simulink model "simulink_caso3_digital"  (R2023a)
settings: Solver=VariableStepAuto  StartTime=0.0  StopTime=10.0  RelTol=1e-3
undefined symbols (not defined in the file): Ad, Aestd, Bd, Bestd, Cd, Cestd, Dd, Destd, K00d, Ts
settings Model: Creator=Agustin  LastModifiedBy=Agustin

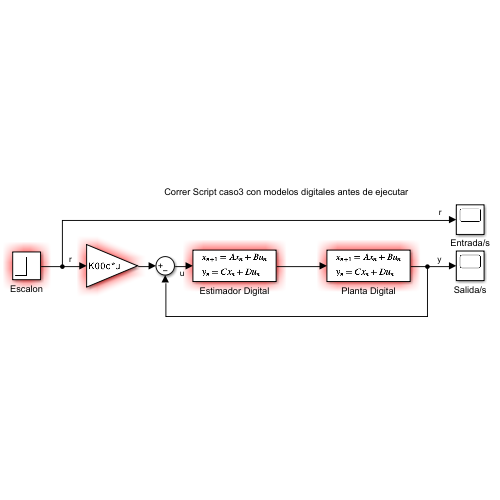
[thumbnail: Simulink's stored preview of the top-level diagram]
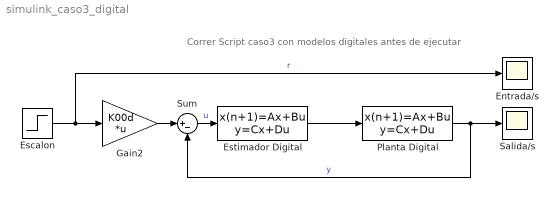
== system simulink_caso3_digital ==
  note: Correr Script caso3 con modelos digitales antes de ejecutar
  Entrada/s : Scope
  Escalon : Step  SampleTime=Ts
  Estimador Digital : DiscreteStateSpace  A=Aestd  B=Bestd  C=Cestd  D=Destd  SampleTime=Ts
  Gain2 : Gain  Gain=K00d  Multiplication=Matrix(K*u)
  Planta Digital : DiscreteStateSpace  A=Ad  B=Bd  C=Cd  D=Dd  SampleTime=Ts
  Salida/s : Scope
  Sum : Sum  Inputs=|+-
  wires:
  Estimador Digital/1 -> Planta Digital/1
  Sum/1 -> Estimador Digital/1  "u"
  Planta Digital/1 -> Salida/s/1, Sum/2  "y"
  Escalon/1 -> Entrada/s/1, Gain2/1  "r"
  Gain2/1 -> Sum/1
